simulink model "sim_Ex2"  (R2022b)
settings: Solver=VariableStepAuto  StartTime=0.0  StopTime=10.0  RelTol=1e-3
libraries: simulink x1
settings Model: Creator=MAAM  LastModifiedBy=MAAM

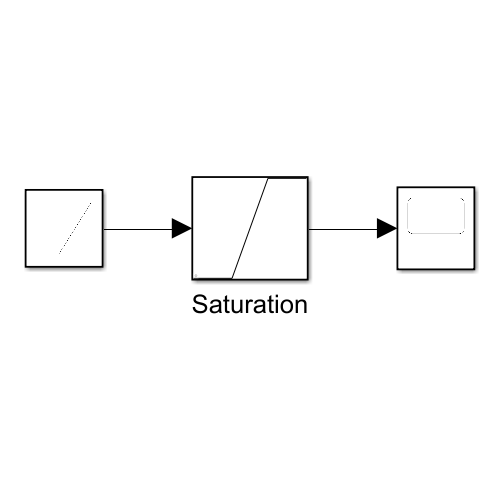
[thumbnail: Simulink's stored preview of the top-level diagram]
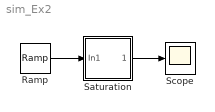
== system sim_Ex2 ==
  Ramp : simulink/Sources/Ramp  slope=2.5  start=0  InitialOutput=-10
  Saturation : Subsystem  mask{Limmits=[-5.0 5.0]}
      mask prompts: Limmits "Limmits [LowerLimmit UpperLimmit]"
      mask init:
      | LowerLimmit = Limmits(1);
      | UpperLimmit = Limmits(2);
      mask DialogControl DescGroupVar Prompt: Saturation Block
      mask DialogControl DescTextVar Prompt: make the output within the limmits
      mask Display: plot([1 2 3 4], [1 1 2 2]);
  Scope : Scope
  wires:
  Ramp/1 -> Saturation/1(In1)
  Saturation/1(Out1) -> Scope/1

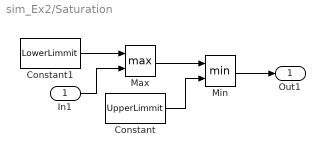
== system sim_Ex2/Saturation ==
  In1 : Inport
  Constant : Constant  Value=UpperLimmit
  Constant1 : Constant  Value=LowerLimmit
  Max : MinMax  Function=max  Inputs=2
  Min : MinMax  Inputs=2
  Out1 : Outport
  wires:
  Min/1 -> Out1/1
  Constant/1 -> Min/2
  Max/1 -> Min/1
  Constant1/1 -> Max/1
  In1/1 -> Max/2
